simulink model "test11"  (R2021a)
settings: Solver=VariableStepAuto  StartTime=0.0  StopTime=8  RelTol=1e-3
model workspace (MAT data in the model file):
  params = climate_p
  params.H = 7.99977069808
  params.A_f = 3100.00026794
  params.A_c = 3299.99999958
  params.minWindows = 0.49999998574
  params.alpha_i = 0.0143839885631
  params.cd_c = 8999.32112543
  params.T_ss = 285
values from neighbouring files (symbols this model uses):
  AR = 20    [test11_script.m]    (also in test11_ws.mat)
libraries: HORTISIM x3
settings Model: SimulationMode=accelerator  OrderedModelArguments=off  Creator=djoroya  LastModifiedBy=djoroya
settings DebuggingCC: UnconnectedInputMsg=none  UnconnectedOutputMsg=none  UnconnectedLineMsg=none

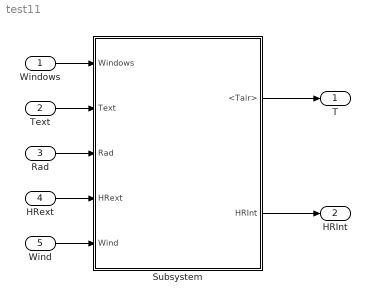
== system test11 ==
  Windows : Inport
  Text : Inport  Port=2
  Rad : Inport  Port=3
  HRext : Inport  Port=4
  Wind : Inport  Port=5
  Subsystem : Subsystem
  T : Outport
  HRInt : Outport  Port=2
  wires:
  Subsystem/1(<Tair>) -> T/1
  Windows/1 -> Subsystem/1(Windows)
  Text/1 -> Subsystem/2(Text)
  Rad/1 -> Subsystem/3(Rad)
  HRext/1 -> Subsystem/4(HRext)
  Wind/1 -> Subsystem/5(Wind)
  Subsystem/2(HRInt) -> HRInt/1

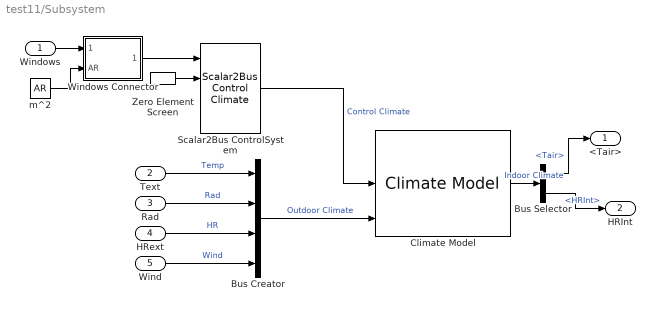
== system test11/Subsystem ==
  Windows : Inport
  Text : Inport  Port=2
  Rad : Inport  Port=3
  HRext : Inport  Port=4
  Wind : Inport  Port=5
  Bus Creator : BusCreator  Inputs=4
  Bus Selector : BusSelector  OutputSignals=Temp.Tair,Gas.HRInt
  Climate Model : HORTISIM/Climate/Models/Climate Model  params=params  x0=cic
      settings: SourceProductName=Horti Simulator
  Scalar2Bus ControlSystem : HORTISIM/Other  Functions/Scalar2Bus  Control Climate  SystemSampleTime=-1  VariantActivationTime=update diagram  Latency=0  AutoFrameSizeCalculation=off
      settings: SourceProductName=Horti Simulator
  Windows Connector : Subsystem
  Zero Element Screen : HORTISIM/Other  Functions/Zero Element Screen  SystemSampleTime=-1  VariantActivationTime=update diagram  Latency=0  AutoFrameSizeCalculation=off
      settings: SourceProductName=Horti Simulator
  m^2 : Constant  Value=AR
  <Tair> : Outport
  HRInt : Outport  Port=2
  wires:
  Scalar2Bus ControlSystem/1 -> Climate Model/2  "Control Climate"
  Climate Model/1 -> Bus Selector/1  "Indoor Climate"
  Bus Creator/1 -> Climate Model/3  "Outdoor Climate"
  Bus Selector/1 -> <Tair>/1  "<Tair>"
  Rad/1 -> Bus Creator/2  "Rad"
  HRext/1 -> Bus Creator/3  "HR"
  Wind/1 -> Bus Creator/4  "Wind"
  Text/1 -> Bus Creator/1  "Temp"
  Bus Selector/2 -> HRInt/1  "<HRInt>"
  Zero Element Screen/1 -> Scalar2Bus ControlSystem/2
  Windows/1 -> Windows Connector/1(value)
  m^2/1 -> Windows Connector/2(AR)
  Windows Connector/1(Windows) -> Scalar2Bus ControlSystem/1

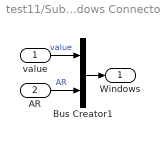
== system test11/Subsystem/Windows Connector ==
  value : Inport
  AR : Inport  Port=2
  Bus Creator1 : BusCreator  Inputs=2
  Windows : Outport
  wires:
  Bus Creator1/1 -> Windows/1
  value/1 -> Bus Creator1/1  "value"
  AR/1 -> Bus Creator1/2  "AR"
